simulink model "FirstDiffTest"  (R2020b)
settings: Solver=VariableStepAuto  StartTime=0.0  StopTime=10.0  RelTol=1e-3
settings Model: Creator=amazi  LastModifiedBy=amazi

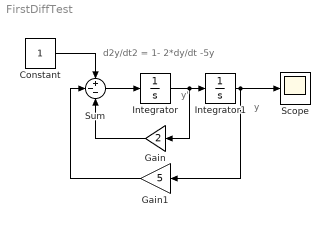
== system FirstDiffTest ==
  note: d2y/dt2 = 1- 2*dy/dt -5y
  note: y
  note: y'
  Constant : Constant
  Gain : Gain  Gain=2
  Gain1 : Gain  Gain=5
  Integrator : Integrator
  Integrator1 : Integrator
  Scope : Scope
  Sum : Sum  Inputs=+--
  wires:
  Integrator/1 -> Integrator1/1, Gain/1
  Integrator1/1 -> Gain1/1, Scope/1
  Constant/1 -> Sum/1
  Gain/1 -> Sum/3
  Gain1/1 -> Sum/2
  Sum/1 -> Integrator/1
